simulink model "BLDC_Motor"  (R2020a)
settings: Solver=VariableStepAuto  StartTime=0.0  StopTime=10.0  RelTol=1e-3
settings Model: Creator=NIKITA  LastModifiedBy=NIKITA

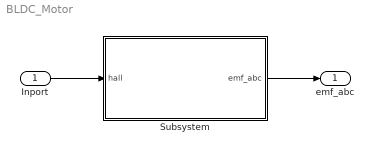
== system BLDC_Motor ==
  Inport : Inport
  "Subsystem " : Subsystem
  emf_abc : Outport
  wires:
  Inport/1 -> "Subsystem "/1(hall)
  "Subsystem "/1(emf_abc) -> emf_abc/1

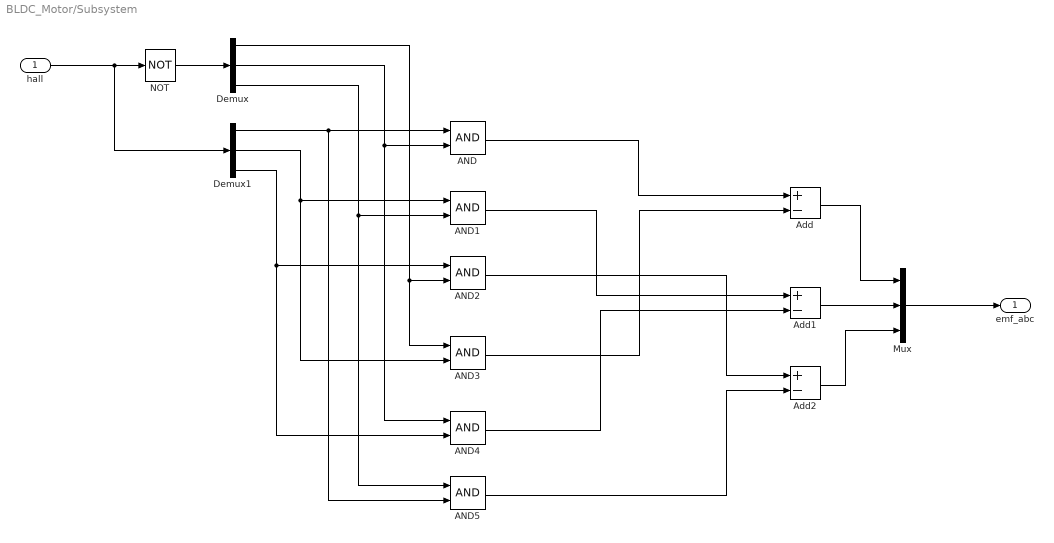
== system BLDC_Motor/Subsystem  ==
  hall : Inport
  AND{,1..5} (6 alike) : Logic  AllPortsSameDT=off  OutDataTypeStr=boolean
  Add : Sum  Inputs=+-
  Add1 : Sum  Inputs=+-
  Add2 : Sum  Inputs=+-
  Demux : Demux  Outputs=3
  Demux1 : Demux  Outputs=3
  Mux : Mux  Inputs=3
  NOT : Logic  Operator=NOT  AllPortsSameDT=off  OutDataTypeStr=boolean
  emf_abc : Outport
  wires:
  Demux/2 -> AND/2, AND4/1
  hall/1 -> Demux1/1, NOT/1
  Mux/1 -> emf_abc/1
  AND/1 -> Add/1
  Demux1/1 -> AND5/2, AND/1
  Demux/3 -> AND1/2, AND5/1
  Add/1 -> Mux/1
  AND5/1 -> Add2/2
  AND1/1 -> Add1/1
  AND3/1 -> Add/2
  Demux1/2 -> AND1/1, AND3/2
  Demux1/3 -> AND4/2, AND2/1
  AND2/1 -> Add2/1
  Demux/1 -> AND3/1, AND2/2
  NOT/1 -> Demux/1
  AND4/1 -> Add1/2
  Add1/1 -> Mux/2
  Add2/1 -> Mux/3
